simulink model "simulink3"  (R2016a)
settings: Solver=VariableStepAuto  StartTime=0.0  StopTime=10.0  RelTol=1e-3
values from neighbouring files (symbols this model uses):
  dc = 5*10^(-2)    (= 0.05)    [pendulum.m]
  g = 9.81    [pendulum.m]
  h = 0.01    [pendulum.m]
  H = 0.010    (= 0.01)    [pendulum.m]
  L = 0.80    (= 0.8)    [pendulum.m]
  r = 0.03    [pendulum.m]
  rho = 3000.0    (= 3000)    [pendulum.m]
  rhos = 7000    [pendulum.m]
  theta0 = pi/2    (= 1.57079632679)    [pendulum.m]
  v0 = 0    [pendulum.m]
  W = 0.010    (= 0.01)    [pendulum.m]
undefined symbols (not defined in the file or in its folder): magnitude
settings Model: Creator=simone  LastModifiedBy=simone

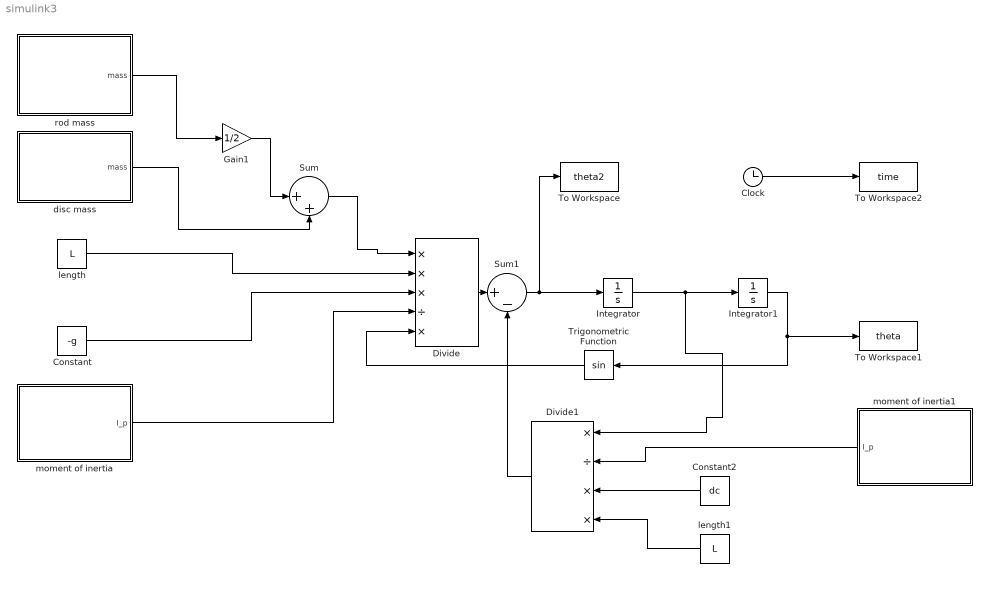
== system simulink3 ==
  Clock : Clock
  Constant : Constant  Value=-g
  Constant2 : Constant  Value=dc
  Divide : Product  Inputs=***/*
  Divide1 : Product  Inputs=*/**
  Gain1 : Gain  Gain=1/2
  Integrator : Integrator  InitialCondition=v0
  Integrator1 : Integrator  InitialCondition=theta0
  Sum : Sum  Inputs=|++
  Sum1 : Sum  Inputs=|+-
  To Workspace : ToWorkspace  VariableName=theta2  SaveFormat=Timeseries  SampleTime=-1
  To Workspace1 : ToWorkspace  VariableName=theta  SaveFormat=Timeseries  SampleTime=-1
  To Workspace2 : ToWorkspace  VariableName=time  SaveFormat=Timeseries  SampleTime=-1
  Trigonometric Function : Trigonometry
  disc mass : Subsystem
  length : Constant  Value=L
  length1 : Constant  Value=L
  moment of inertia : Subsystem
  moment of inertia1 : Subsystem
  rod mass : Subsystem
  wires:
  rod mass/1("mass ") -> Gain1/1
  Gain1/1 -> Sum/1
  disc mass/1(mass) -> Sum/2
  Sum/1 -> Divide/1
  length/1 -> Divide/2
  Constant/1 -> Divide/3
  moment of inertia/1("I_p ") -> Divide/4
  Integrator1/1 -> To Workspace1/1, Trigonometric Function/1
  Trigonometric Function/1 -> Divide/5
  Sum1/1 -> To Workspace/1, Integrator/1
  Clock/1 -> To Workspace2/1
  Divide/1 -> Sum1/1
  Constant2/1 -> Divide1/3
  moment of inertia1/1("I_p ") -> Divide1/2
  Divide1/1 -> Sum1/2
  Integrator/1 -> Divide1/1, Integrator1/1
  length1/1 -> Divide1/4

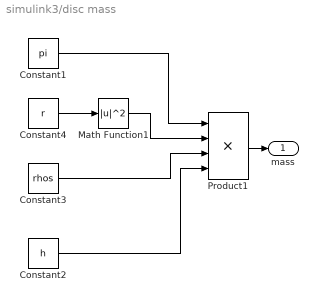
== system simulink3/disc mass ==
  Constant1 : Constant  Value=pi
  Constant2 : Constant  Value=h
  Constant3 : Constant  Value=rhos
  Constant4 : Constant  Value=r
  Math Function1 : Math  Operator=magnitude^2  SaturateOnIntegerOverflow=on
  Product1 : Product  Inputs=4
  mass : Outport
  wires:
  Constant3/1 -> Product1/3
  Constant2/1 -> Product1/4
  Math Function1/1 -> Product1/2
  Product1/1 -> mass/1
  Constant4/1 -> Math Function1/1
  Constant1/1 -> Product1/1

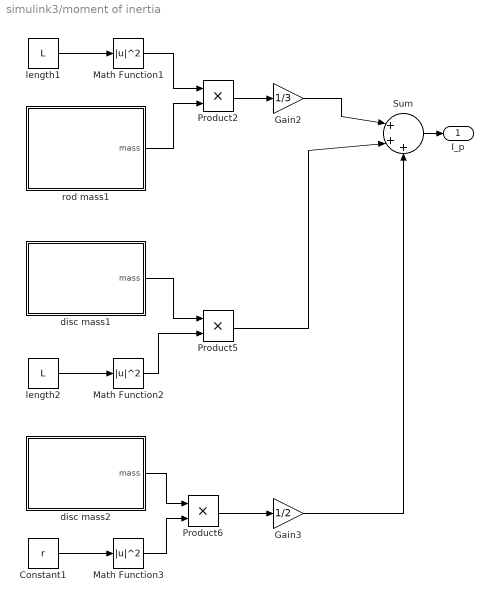
== system simulink3/moment of inertia ==
  Constant1 : Constant  Value=r
  Gain2 : Gain  Gain=1/3
  Gain3 : Gain  Gain=1/2
  Math Function1 : Math  Operator=magnitude^2  SaturateOnIntegerOverflow=on
  Math Function2 : Math  Operator=magnitude^2  SaturateOnIntegerOverflow=on
  Math Function3 : Math  Operator=magnitude^2  SaturateOnIntegerOverflow=on
  Product2 : Product
  Product5 : Product
  Product6 : Product
  Sum : Sum  Inputs=|+++
  disc mass1 : Subsystem
  disc mass2 : Subsystem
  length1 : Constant  Value=L
  length2 : Constant  Value=L
  rod mass1 : Subsystem
  "I_p " : Outport
  wires:
  Math Function2/1 -> Product5/2
  Product5/1 -> Sum/2
  Gain3/1 -> Sum/3
  length2/1 -> Math Function2/1
  Product2/1 -> Gain2/1
  Gain2/1 -> Sum/1
  Constant1/1 -> Math Function3/1
  Math Function1/1 -> Product2/1
  Sum/1 -> "I_p "/1
  length1/1 -> Math Function1/1
  disc mass1/1(mass) -> Product5/1
  Math Function3/1 -> Product6/2
  rod mass1/1("mass ") -> Product2/2
  disc mass2/1(mass) -> Product6/1
  Product6/1 -> Gain3/1

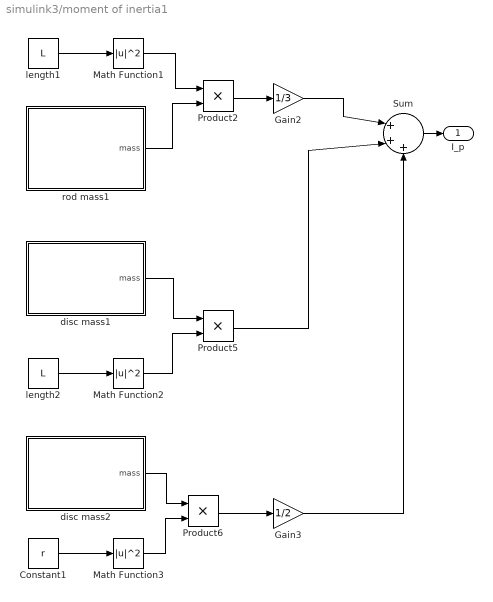
== system simulink3/moment of inertia1 ==
  Constant1 : Constant  Value=r
  Gain2 : Gain  Gain=1/3
  Gain3 : Gain  Gain=1/2
  Math Function1 : Math  Operator=magnitude^2  SaturateOnIntegerOverflow=on
  Math Function2 : Math  Operator=magnitude^2  SaturateOnIntegerOverflow=on
  Math Function3 : Math  Operator=magnitude^2  SaturateOnIntegerOverflow=on
  Product2 : Product
  Product5 : Product
  Product6 : Product
  Sum : Sum  Inputs=|+++
  disc mass1 : Subsystem
  disc mass2 : Subsystem
  length1 : Constant  Value=L
  length2 : Constant  Value=L
  rod mass1 : Subsystem
  "I_p " : Outport
  wires:
  Math Function2/1 -> Product5/2
  Product5/1 -> Sum/2
  Gain3/1 -> Sum/3
  length2/1 -> Math Function2/1
  Product2/1 -> Gain2/1
  Gain2/1 -> Sum/1
  Constant1/1 -> Math Function3/1
  Math Function1/1 -> Product2/1
  Sum/1 -> "I_p "/1
  length1/1 -> Math Function1/1
  disc mass1/1(mass) -> Product5/1
  Math Function3/1 -> Product6/2
  rod mass1/1("mass ") -> Product2/2
  disc mass2/1(mass) -> Product6/1
  Product6/1 -> Gain3/1

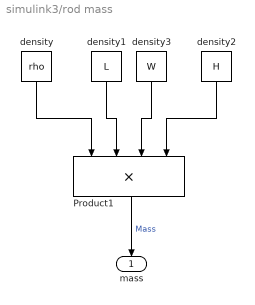
== system simulink3/rod mass ==
  Product1 : Product  Inputs=4
  density : Constant  Value=rho
  density1 : Constant  Value=L
  density2 : Constant  Value=H
  density3 : Constant  Value=W
  "mass " : Outport
  wires:
  density2/1 -> Product1/4
  density/1 -> Product1/1
  density3/1 -> Product1/3
  density1/1 -> Product1/2
  Product1/1 -> "mass "/1  "Mass"

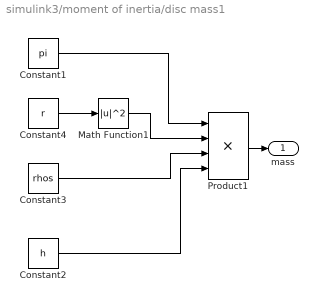
== system simulink3/moment of inertia/disc mass1 ==
  Constant1 : Constant  Value=pi
  Constant2 : Constant  Value=h
  Constant3 : Constant  Value=rhos
  Constant4 : Constant  Value=r
  Math Function1 : Math  Operator=magnitude^2  SaturateOnIntegerOverflow=on
  Product1 : Product  Inputs=4
  mass : Outport
  wires:
  Constant3/1 -> Product1/3
  Constant2/1 -> Product1/4
  Math Function1/1 -> Product1/2
  Product1/1 -> mass/1
  Constant4/1 -> Math Function1/1
  Constant1/1 -> Product1/1

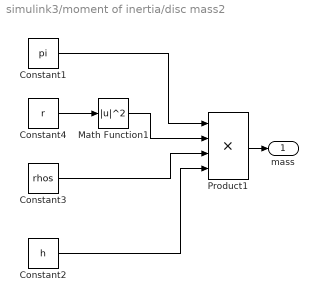
== system simulink3/moment of inertia/disc mass2 ==
  Constant1 : Constant  Value=pi
  Constant2 : Constant  Value=h
  Constant3 : Constant  Value=rhos
  Constant4 : Constant  Value=r
  Math Function1 : Math  Operator=magnitude^2  SaturateOnIntegerOverflow=on
  Product1 : Product  Inputs=4
  mass : Outport
  wires:
  Constant3/1 -> Product1/3
  Constant2/1 -> Product1/4
  Math Function1/1 -> Product1/2
  Product1/1 -> mass/1
  Constant4/1 -> Math Function1/1
  Constant1/1 -> Product1/1

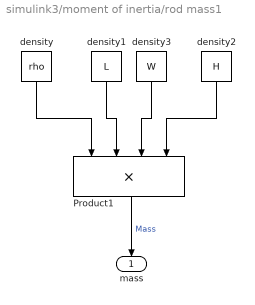
== system simulink3/moment of inertia/rod mass1 ==
  Product1 : Product  Inputs=4
  density : Constant  Value=rho
  density1 : Constant  Value=L
  density2 : Constant  Value=H
  density3 : Constant  Value=W
  "mass " : Outport
  wires:
  density2/1 -> Product1/4
  density/1 -> Product1/1
  density3/1 -> Product1/3
  density1/1 -> Product1/2
  Product1/1 -> "mass "/1  "Mass"

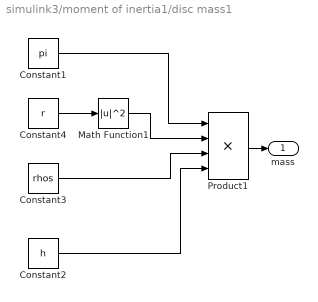
== system simulink3/moment of inertia1/disc mass1 ==
  Constant1 : Constant  Value=pi
  Constant2 : Constant  Value=h
  Constant3 : Constant  Value=rhos
  Constant4 : Constant  Value=r
  Math Function1 : Math  Operator=magnitude^2  SaturateOnIntegerOverflow=on
  Product1 : Product  Inputs=4
  mass : Outport
  wires:
  Constant3/1 -> Product1/3
  Constant2/1 -> Product1/4
  Math Function1/1 -> Product1/2
  Product1/1 -> mass/1
  Constant4/1 -> Math Function1/1
  Constant1/1 -> Product1/1

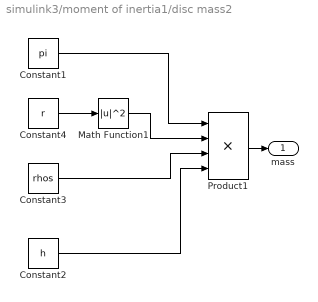
== system simulink3/moment of inertia1/disc mass2 ==
  Constant1 : Constant  Value=pi
  Constant2 : Constant  Value=h
  Constant3 : Constant  Value=rhos
  Constant4 : Constant  Value=r
  Math Function1 : Math  Operator=magnitude^2  SaturateOnIntegerOverflow=on
  Product1 : Product  Inputs=4
  mass : Outport
  wires:
  Constant3/1 -> Product1/3
  Constant2/1 -> Product1/4
  Math Function1/1 -> Product1/2
  Product1/1 -> mass/1
  Constant4/1 -> Math Function1/1
  Constant1/1 -> Product1/1

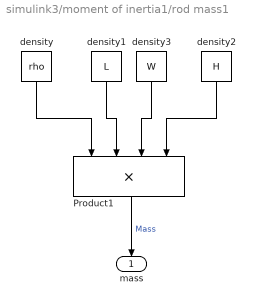
== system simulink3/moment of inertia1/rod mass1 ==
  Product1 : Product  Inputs=4
  density : Constant  Value=rho
  density1 : Constant  Value=L
  density2 : Constant  Value=H
  density3 : Constant  Value=W
  "mass " : Outport
  wires:
  density2/1 -> Product1/4
  density/1 -> Product1/1
  density3/1 -> Product1/3
  density1/1 -> Product1/2
  Product1/1 -> "mass "/1  "Mass"
